simulink model "symulacja_MP"  (R2019b)
settings: Solver=VariableStepAuto  StartTime=0.0  StopTime=50  RelTol=1e-3
values from neighbouring files (symbols this model uses):
  d = 1    [lab8.m]
  Kr = 0.3    [lab8.m]
  m = 0.5    [lab8.m]
  T_o = 0.1    [lab8.m]
  y_sp = 0.1    [lab8.m]
settings Model: Creator=kacpe  LastModifiedBy=kacpe

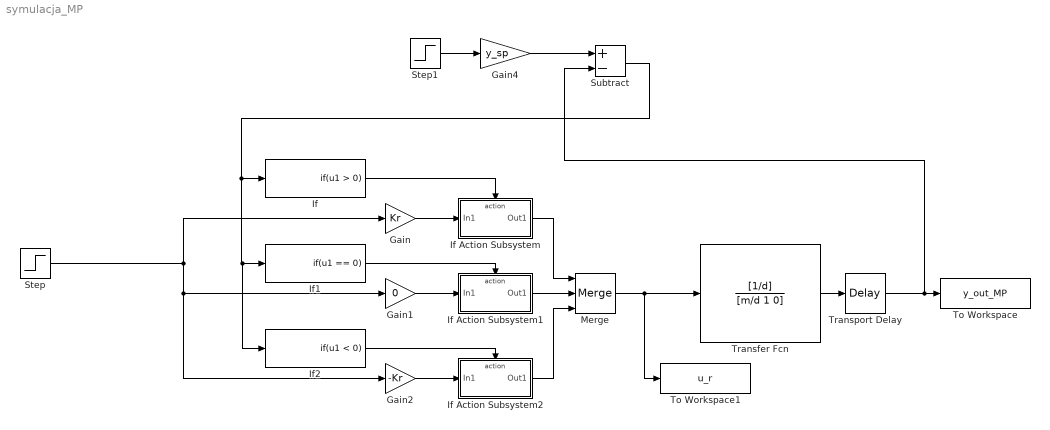
== system symulacja_MP ==
  Gain : Gain  Gain=Kr
  Gain1 : Gain  Gain=0
  Gain2 : Gain  Gain=-Kr
  Gain4 : Gain  Gain=y_sp
  If : If  ShowElse=off
  If Action Subsystem : Subsystem  TreatAsAtomicUnit=on
  If Action Subsystem1 : Subsystem  TreatAsAtomicUnit=on
  If Action Subsystem2 : Subsystem  TreatAsAtomicUnit=on
  If1 : If  IfExpression=u1 == 0  ShowElse=off
  If2 : If  IfExpression=u1 < 0  ShowElse=off
  Merge : Merge  Inputs=3
  Step : Step  SampleTime=0
  Step1 : Step  SampleTime=0
  Subtract : Sum  Inputs=+-
  To Workspace : ToWorkspace  VariableName=y_out_MP  SampleTime=-1
  To Workspace1 : ToWorkspace  VariableName=u_r  SampleTime=-1
  Transfer Fcn : TransferFcn  Numerator=[1/d]  Denominator=[m/d 1 0]
  Transport Delay : TransportDelay  DelayTime=T_o
  wires:
  If/1 -> If Action Subsystem/Action
  If1/1 -> If Action Subsystem1/Action
  If2/1 -> If Action Subsystem2/Action
  Gain1/1 -> If Action Subsystem1/1(In1)
  Gain/1 -> If Action Subsystem/1(In1)
  Gain2/1 -> If Action Subsystem2/1(In1)
  Step/1 -> Gain2/1, Gain1/1, Gain/1
  Merge/1 -> To Workspace1/1, Transfer Fcn/1
  Transfer Fcn/1 -> Transport Delay/1
  If Action Subsystem1/1(Out1) -> Merge/2
  If Action Subsystem/1(Out1) -> Merge/1
  If Action Subsystem2/1(Out1) -> Merge/3
  Transport Delay/1 -> To Workspace/1, Subtract/2
  Step1/1 -> Gain4/1
  Gain4/1 -> Subtract/1
  Subtract/1 -> If2/1, If1/1, If/1

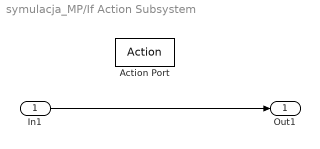
== system symulacja_MP/If Action Subsystem ==
  In1 : Inport
  Action Port : ActionPort  ActionPortLabel=if(u1 > 0)
  Out1 : Outport
  wires:
  In1/1 -> Out1/1

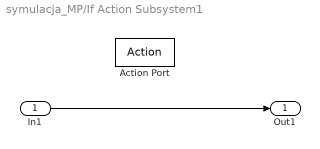
== system symulacja_MP/If Action Subsystem1 ==
  In1 : Inport
  Action Port : ActionPort  ActionPortLabel=if(u1 == 0)
  Out1 : Outport
  wires:
  In1/1 -> Out1/1

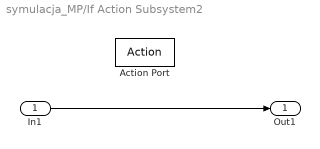
== system symulacja_MP/If Action Subsystem2 ==
  In1 : Inport
  Action Port : ActionPort  ActionPortLabel=if(u1 < 0)
  Out1 : Outport
  wires:
  In1/1 -> Out1/1
